simulink model "CM010A_GmT1xxMcuCfg"  (R2013b)
settings: Solver=FixedStepDiscrete  SolverMode=SingleTasking  StartTime=0.0  StopTime=0.05  RelTol=1e-3
undefined symbols (not defined in the file): BATTVLTGSCAGFAC_ULS_F32, BATTVLTGSWD1SCAGFAC_ULS_F32, BATTVLTGSWD2SCAGFAC_ULS_F32, sigbuilder_block
libraries: CM010A_GmT1xxMcuCfg_ModelLibrary x68, simulink x31
(part 2 of 3)

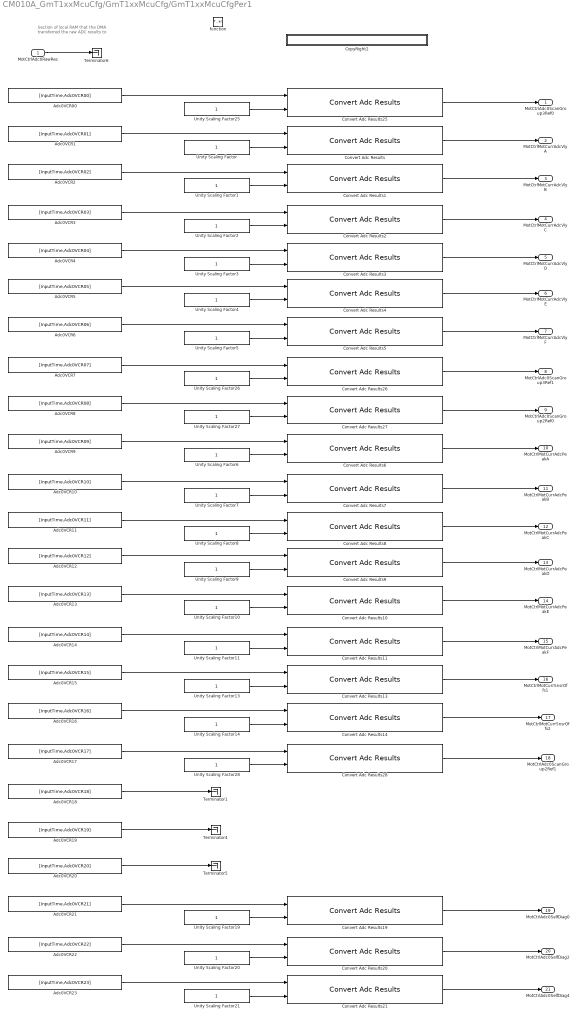
== system CM010A_GmT1xxMcuCfg/GmT1xxMcuCfg/GmT1xxMcuCfgPer1 ==
  note: Section of local RAM that the
      | DMA transferred the raw
      | ADC results to
  MotCtrlAdc0RawRes : Inport
  function : TriggerPort  TriggerType=function-call
  Adc0VCR00 : FromWorkspace  RequirementInfo={'linktype_rmi_doors' '000089ae (/ESG Group/FDD Module Requirements/ES FDDs/ES-50A DigMSB Allegro A1331)' '#ES50A_543' 'true' '3.3.2.2.0-1 The DigMSB Allegro 1331 Function shall indicate the integrity' '' } %GIDa_3972507b_7f96_4457_a8c5_9a064fa93529  VariableName=[InputTime,Adc0VCR00]  Interpolate=off  OutputAfterFinalValue=Holding final value
  Adc0VCR1 : FromWorkspace  RequirementInfo={'linktype_rmi_doors' '000089ae (/ESG Group/FDD Module Requirements/ES FDDs/ES-50A DigMSB Allegro A1331)' '#ES50A_543' 'true' '3.3.2.2.0-1 The DigMSB Allegro 1331 Function shall indicate the integrity' '' } %GIDa_8df7c0a1_9c18_4830_b8c1_52194c851c06  VariableName=[InputTime,Adc0VCR01]  Interpolate=off  OutputAfterFinalValue=Holding final value
  Adc0VCR10 : FromWorkspace  RequirementInfo={'linktype_rmi_doors' '000089ae (/ESG Group/FDD Module Requirements/ES FDDs/ES-50A DigMSB Allegro A1331)' '#ES50A_543' 'true' '3.3.2.2.0-1 The DigMSB Allegro 1331 Function shall indicate the integrity' '' } %GIDa_ced24115_ee0e_48d7_a1c5_ed88c1ec89e4  VariableName=[InputTime,Adc0VCR10]  Interpolate=off  OutputAfterFinalValue=Holding final value
  Adc0VCR11 : FromWorkspace  RequirementInfo={'linktype_rmi_doors' '000089ae (/ESG Group/FDD Module Requirements/ES FDDs/ES-50A DigMSB Allegro A1331)' '#ES50A_543' 'true' '3.3.2.2.0-1 The DigMSB Allegro 1331 Function shall indicate the integrity' '' } %GIDa_db2b065f_31fb_41aa_814a_e5cf8b57cff8  VariableName=[InputTime,Adc0VCR11]  Interpolate=off  OutputAfterFinalValue=Holding final value
  Adc0VCR12 : FromWorkspace  RequirementInfo={'linktype_rmi_doors' '000089ae (/ESG Group/FDD Module Requirements/ES FDDs/ES-50A DigMSB Allegro A1331)' '#ES50A_543' 'true' '3.3.2.2.0-1 The DigMSB Allegro 1331 Function shall indicate the integrity' '' } %GIDa_d2596e36_6e68_4a9e_ad4d_131e4edbf304  VariableName=[InputTime,Adc0VCR12]  Interpolate=off  OutputAfterFinalValue=Holding final value
  Adc0VCR13 : FromWorkspace  RequirementInfo={'linktype_rmi_doors' '000089ae (/ESG Group/FDD Module Requirements/ES FDDs/ES-50A DigMSB Allegro A1331)' '#ES50A_543' 'true' '3.3.2.2.0-1 The DigMSB Allegro 1331 Function shall indicate the integrity' '' } %GIDa_588422b8_9a00_4d95_845d_3e9dda5825e6  VariableName=[InputTime,Adc0VCR13]  Interpolate=off  OutputAfterFinalValue=Holding final value
  Adc0VCR14 : FromWorkspace  RequirementInfo={'linktype_rmi_doors' '000089ae (/ESG Group/FDD Module Requirements/ES FDDs/ES-50A DigMSB Allegro A1331)' '#ES50A_543' 'true' '3.3.2.2.0-1 The DigMSB Allegro 1331 Function shall indicate the integrity' '' } %GIDa_7f782811_0c4f_4bde_8d07_b52392360608  VariableName=[InputTime,Adc0VCR14]  Interpolate=off  OutputAfterFinalValue=Holding final value
  Adc0VCR15 : FromWorkspace  RequirementInfo={'linktype_rmi_doors' '000089ae (/ESG Group/FDD Module Requirements/ES FDDs/ES-50A DigMSB Allegro A1331)' '#ES50A_543' 'true' '3.3.2.2.0-1 The DigMSB Allegro 1331 Function shall indicate the integrity' '' } %GIDa_e774656f_bc2d_46bf_a587_e8a39f34598c  VariableName=[InputTime,Adc0VCR15]  Interpolate=off  OutputAfterFinalValue=Holding final value
  Adc0VCR16 : FromWorkspace  RequirementInfo={'linktype_rmi_doors' '000089ae (/ESG Group/FDD Module Requirements/ES FDDs/ES-50A DigMSB Allegro A1331)' '#ES50A_543' 'true' '3.3.2.2.0-1 The DigMSB Allegro 1331 Function shall indicate the integrity' '' } %GIDa_f44d6d24_48ad_4518_886b_ff8438f6312a  VariableName=[InputTime,Adc0VCR16]  Interpolate=off  OutputAfterFinalValue=Holding final value
  Adc0VCR17 : FromWorkspace  RequirementInfo={'linktype_rmi_doors' '000089ae (/ESG Group/FDD Module Requirements/ES FDDs/ES-50A DigMSB Allegro A1331)' '#ES50A_543' 'true' '3.3.2.2.0-1 The DigMSB Allegro 1331 Function shall indicate the integrity' '' } %GIDa_4675bda8_e067_4190_b347_8310ec6ff6c1  VariableName=[InputTime,Adc0VCR17]  Interpolate=off  OutputAfterFinalValue=Holding final value
  Adc0VCR18 : FromWorkspace  RequirementInfo={'linktype_rmi_doors' '000089ae (/ESG Group/FDD Module Requirements/ES FDDs/ES-50A DigMSB Allegro A1331)' '#ES50A_543' 'true' '3.3.2.2.0-1 The DigMSB Allegro 1331 Function shall indicate the integrity' '' } %GIDa_5aa89b95_9bd8_4248_9c0f_b5e881e1f776  VariableName=[InputTime,Adc0VCR18]  Interpolate=off  OutputAfterFinalValue=Holding final value
  Adc0VCR19 : FromWorkspace  RequirementInfo={'linktype_rmi_doors' '000089ae (/ESG Group/FDD Module Requirements/ES FDDs/ES-50A DigMSB Allegro A1331)' '#ES50A_543' 'true' '3.3.2.2.0-1 The DigMSB Allegro 1331 Function shall indicate the integrity' '' } %GIDa_d11aca7d_abc9_46a3_9261_b33926c9d20c  VariableName=[InputTime,Adc0VCR19]  Interpolate=off  OutputAfterFinalValue=Holding final value
  Adc0VCR2 : FromWorkspace  RequirementInfo={'linktype_rmi_doors' '000089ae (/ESG Group/FDD Module Requirements/ES FDDs/ES-50A DigMSB Allegro A1331)' '#ES50A_543' 'true' '3.3.2.2.0-1 The DigMSB Allegro 1331 Function shall indicate the integrity' '' } %GIDa_f6b758eb_17b3_4646_850a_50046f5107be  VariableName=[InputTime,Adc0VCR02]  Interpolate=off  OutputAfterFinalValue=Holding final value
  Adc0VCR20 : FromWorkspace  RequirementInfo={'linktype_rmi_doors' '000089ae (/ESG Group/FDD Module Requirements/ES FDDs/ES-50A DigMSB Allegro A1331)' '#ES50A_543' 'true' '3.3.2.2.0-1 The DigMSB Allegro 1331 Function shall indicate the integrity' '' } %GIDa_43dd3eb4_cf09_4920_adef_b45211e1cdfd  VariableName=[InputTime,Adc0VCR20]  Interpolate=off  OutputAfterFinalValue=Holding final value
  Adc0VCR21 : FromWorkspace  RequirementInfo={'linktype_rmi_doors' '000089ae (/ESG Group/FDD Module Requirements/ES FDDs/ES-50A DigMSB Allegro A1331)' '#ES50A_543' 'true' '3.3.2.2.0-1 The DigMSB Allegro 1331 Function shall indicate the integrity' '' } %GIDa_6a9825af_16e5_42b4_afa2_2084b93d0a1b  VariableName=[InputTime,Adc0VCR21]  Interpolate=off  OutputAfterFinalValue=Holding final value
  Adc0VCR22 : FromWorkspace  RequirementInfo={'linktype_rmi_doors' '000089ae (/ESG Group/FDD Module Requirements/ES FDDs/ES-50A DigMSB Allegro A1331)' '#ES50A_543' 'true' '3.3.2.2.0-1 The DigMSB Allegro 1331 Function shall indicate the integrity' '' } %GIDa_29a8826e_1cf3_4183_be72_0450154b9da2  VariableName=[InputTime,Adc0VCR22]  Interpolate=off  OutputAfterFinalValue=Holding final value
  Adc0VCR23 : FromWorkspace  RequirementInfo={'linktype_rmi_doors' '000089ae (/ESG Group/FDD Module Requirements/ES FDDs/ES-50A DigMSB Allegro A1331)' '#ES50A_543' 'true' '3.3.2.2.0-1 The DigMSB Allegro 1331 Function shall indicate the integrity' '' } %GIDa_8d461b89_add0_42d0_84ba_8109d18c3aa6  VariableName=[InputTime,Adc0VCR23]  Interpolate=off  OutputAfterFinalValue=Holding final value
  Adc0VCR3 : FromWorkspace  RequirementInfo={'linktype_rmi_doors' '000089ae (/ESG Group/FDD Module Requirements/ES FDDs/ES-50A DigMSB Allegro A1331)' '#ES50A_543' 'true' '3.3.2.2.0-1 The DigMSB Allegro 1331 Function shall indicate the integrity' '' } %GIDa_7f5e4bfd_0dc0_4fd2_91a2_992d3fd35db3  VariableName=[InputTime,Adc0VCR03]  Interpolate=off  OutputAfterFinalValue=Holding final value
  Adc0VCR4 : FromWorkspace  RequirementInfo={'linktype_rmi_doors' '000089ae (/ESG Group/FDD Module Requirements/ES FDDs/ES-50A DigMSB Allegro A1331)' '#ES50A_543' 'true' '3.3.2.2.0-1 The DigMSB Allegro 1331 Function shall indicate the integrity' '' } %GIDa_65871648_6683_4b6d_aff0_bffed2640892  VariableName=[InputTime,Adc0VCR04]  Interpolate=off  OutputAfterFinalValue=Holding final value
  Adc0VCR5 : FromWorkspace  RequirementInfo={'linktype_rmi_doors' '000089ae (/ESG Group/FDD Module Requirements/ES FDDs/ES-50A DigMSB Allegro A1331)' '#ES50A_543' 'true' '3.3.2.2.0-1 The DigMSB Allegro 1331 Function shall indicate the integrity' '' } %GIDa_516afef0_9b4d_432f_89dd_5f746eb09d49  VariableName=[InputTime,Adc0VCR05]  Interpolate=off  OutputAfterFinalValue=Holding final value
  Adc0VCR6 : FromWorkspace  RequirementInfo={'linktype_rmi_doors' '000089ae (/ESG Group/FDD Module Requirements/ES FDDs/ES-50A DigMSB Allegro A1331)' '#ES50A_543' 'true' '3.3.2.2.0-1 The DigMSB Allegro 1331 Function shall indicate the integrity' '' } %GIDa_384fee31_75ed_46f0_a695_7bc76fa48fd4  VariableName=[InputTime,Adc0VCR06]  Interpolate=off  OutputAfterFinalValue=Holding final value
  Adc0VCR7 : FromWorkspace  RequirementInfo={'linktype_rmi_doors' '000089ae (/ESG Group/FDD Module Requirements/ES FDDs/ES-50A DigMSB Allegro A1331)' '#ES50A_543' 'true' '3.3.2.2.0-1 The DigMSB Allegro 1331 Function shall indicate the integrity' '' } %GIDa_8c377a38_d7bd_42ca_a29f_4b53229cfff5  VariableName=[InputTime,Adc0VCR07]  Interpolate=off  OutputAfterFinalValue=Holding final value
  Adc0VCR8 : FromWorkspace  RequirementInfo={'linktype_rmi_doors' '000089ae (/ESG Group/FDD Module Requirements/ES FDDs/ES-50A DigMSB Allegro A1331)' '#ES50A_543' 'true' '3.3.2.2.0-1 The DigMSB Allegro 1331 Function shall indicate the integrity' '' } %GIDa_dae074de_385b_4abf_a24d_4693de33c827  VariableName=[InputTime,Adc0VCR08]  Interpolate=off  OutputAfterFinalValue=Holding final value
  Adc0VCR9 : FromWorkspace  RequirementInfo={'linktype_rmi_doors' '000089ae (/ESG Group/FDD Module Requirements/ES FDDs/ES-50A DigMSB Allegro A1331)' '#ES50A_543' 'true' '3.3.2.2.0-1 The DigMSB Allegro 1331 Function shall indicate the integrity' '' } %GIDa_c1adce1a_ec60_4755_95aa_f8dbf63dfb59  VariableName=[InputTime,Adc0VCR09]  Interpolate=off  OutputAfterFinalValue=Holding final value
  Convert Adc Results{,1..11,13..14,19..21,25..28} (21 alike) : CM010A_GmT1xxMcuCfg_ModelLibrary/Convert Adc Results
  CopyRight2 : Subsystem  Description=|  mask(Copyright Information){none=on}
      | Copyright info block.                                               
      |                                                                     
      | Place copyright information at the top of every subsystem in design.
      mask prompts: none "No parameters"
      mask help: Place copyright information at the top of every subsystem in design.
      mask Display:
      | NxtrConf = 'Nexteer Confidential';
      | 
      | sys = bdroot; %handle for the current model ("system")
      | first = get_param(sys,'Created');
      | first = first(end-3:end);  %year is last four digits
      | 
      | last = get_param(sys,'LastModifiedDate');
      | if isempty(last)
      |     last = datestr(now,'yyyy');
      | else
      |     last = last(end-3:end);
      | end
      | 
      | if strcmp(first,last)
      |     fprintf('%s -- Copyright %s Nexteer',NxtrConf,first)
      | else
      |     fprintf('%s -- %s%s- %s Nexteer',NxtrConf,char(169),first,last)
      | end
  Terminator{1,4..6} (4 alike) : Terminator
  Unity Scaling Factor{,1..11,13..14,19..21,25..28} (21 alike) : Constant  OutDataTypeStr=single
  MotCtrlAdc0ScanGroup3Ref0 : Outport
  MotCtrlMotCurrAdcVlyA : Outport  Port=2
  MotCtrlMotCurrAdcVlyB : Outport  Port=3
  MotCtrlMotCurrAdcVlyC : Outport  Port=4
  MotCtrlMotCurrAdcVlyD : Outport  Port=5
  MotCtrlMotCurrAdcVlyE : Outport  Port=6
  MotCtrlMotCurrAdcVlyF : Outport  Port=7
  MotCtrlAdc0ScanGroup3Ref1 : Outport  Port=8
  MotCtrlAdc0ScanGroup2Ref0 : Outport  Port=9
  MotCtrlMotCurrAdcPeakA : Outport  Port=10
  MotCtrlMotCurrAdcPeakB : Outport  Port=11
  MotCtrlMotCurrAdcPeakC : Outport  Port=12
  MotCtrlMotCurrAdcPeakD : Outport  Port=13
  MotCtrlMotCurrAdcPeakE : Outport  Port=14
  MotCtrlMotCurrAdcPeakF : Outport  Port=15
  MotCtrlMotCurrSnsrOffs1 : Outport  Port=16
  MotCtrlMotCurrSnsrOffs2 : Outport  Port=17
  MotCtrlAdc0ScanGroup2Ref1 : Outport  Port=18
  MotCtrlAdc0SelfDiag0 : Outport  Port=19
  MotCtrlAdc0SelfDiag2 : Outport  Port=20
  MotCtrlAdc0SelfDiag4 : Outport  Port=21
  wires:
  Unity Scaling Factor/1 -> Convert Adc Results/2
  Unity Scaling Factor1/1 -> Convert Adc Results1/2
  Unity Scaling Factor2/1 -> Convert Adc Results2/2
  Unity Scaling Factor3/1 -> Convert Adc Results3/2
  Unity Scaling Factor4/1 -> Convert Adc Results4/2
  Unity Scaling Factor5/1 -> Convert Adc Results5/2
  Unity Scaling Factor6/1 -> Convert Adc Results6/2
  Unity Scaling Factor7/1 -> Convert Adc Results7/2
  Unity Scaling Factor8/1 -> Convert Adc Results8/2
  Unity Scaling Factor9/1 -> Convert Adc Results9/2
  Unity Scaling Factor10/1 -> Convert Adc Results10/2
  Unity Scaling Factor11/1 -> Convert Adc Results11/2
  Unity Scaling Factor13/1 -> Convert Adc Results13/2
  Unity Scaling Factor14/1 -> Convert Adc Results14/2
  Adc0VCR21/1 -> Convert Adc Results19/1
  Unity Scaling Factor19/1 -> Convert Adc Results19/2
  Adc0VCR22/1 -> Convert Adc Results20/1
  Unity Scaling Factor20/1 -> Convert Adc Results20/2
  Adc0VCR23/1 -> Convert Adc Results21/1
  Unity Scaling Factor21/1 -> Convert Adc Results21/2
  Convert Adc Results2/1 -> MotCtrlMotCurrAdcVlyC/1
  Convert Adc Results3/1 -> MotCtrlMotCurrAdcVlyD/1
  Convert Adc Results4/1 -> MotCtrlMotCurrAdcVlyE/1
  Convert Adc Results5/1 -> MotCtrlMotCurrAdcVlyF/1
  Convert Adc Results6/1 -> MotCtrlMotCurrAdcPeakA/1
  Convert Adc Results7/1 -> MotCtrlMotCurrAdcPeakB/1
  Convert Adc Results8/1 -> MotCtrlMotCurrAdcPeakC/1
  Convert Adc Results9/1 -> MotCtrlMotCurrAdcPeakD/1
  Convert Adc Results10/1 -> MotCtrlMotCurrAdcPeakE/1
  Convert Adc Results11/1 -> MotCtrlMotCurrAdcPeakF/1
  Convert Adc Results13/1 -> MotCtrlMotCurrSnsrOffs1/1
  Convert Adc Results14/1 -> MotCtrlMotCurrSnsrOffs2/1
  Convert Adc Results19/1 -> MotCtrlAdc0SelfDiag0/1
  Convert Adc Results20/1 -> MotCtrlAdc0SelfDiag2/1
  Convert Adc Results21/1 -> MotCtrlAdc0SelfDiag4/1
  Adc0VCR20/1 -> Terminator5/1
  Adc0VCR19/1 -> Terminator4/1
  MotCtrlAdc0RawRes/1 -> Terminator6/1
  Unity Scaling Factor25/1 -> Convert Adc Results25/2
  Convert Adc Results25/1 -> MotCtrlAdc0ScanGroup3Ref0/1
  Unity Scaling Factor26/1 -> Convert Adc Results26/2
  Convert Adc Results26/1 -> MotCtrlAdc0ScanGroup3Ref1/1
  Unity Scaling Factor27/1 -> Convert Adc Results27/2
  Convert Adc Results27/1 -> MotCtrlAdc0ScanGroup2Ref0/1
  Unity Scaling Factor28/1 -> Convert Adc Results28/2
  Convert Adc Results28/1 -> MotCtrlAdc0ScanGroup2Ref1/1
  Adc0VCR1/1 -> Convert Adc Results/1
  Adc0VCR7/1 -> Convert Adc Results26/1
  Adc0VCR8/1 -> Convert Adc Results27/1
  Adc0VCR00/1 -> Convert Adc Results25/1
  Convert Adc Results1/1 -> MotCtrlMotCurrAdcVlyB/1
  Convert Adc Results/1 -> MotCtrlMotCurrAdcVlyA/1
  Adc0VCR14/1 -> Convert Adc Results11/1
  Adc0VCR13/1 -> Convert Adc Results10/1
  Adc0VCR12/1 -> Convert Adc Results9/1
  Adc0VCR11/1 -> Convert Adc Results8/1
  Adc0VCR10/1 -> Convert Adc Results7/1
  Adc0VCR9/1 -> Convert Adc Results6/1
  Adc0VCR6/1 -> Convert Adc Results5/1
  Adc0VCR5/1 -> Convert Adc Results4/1
  Adc0VCR4/1 -> Convert Adc Results3/1
  Adc0VCR3/1 -> Convert Adc Results2/1
  Adc0VCR2/1 -> Convert Adc Results1/1
  Adc0VCR15/1 -> Convert Adc Results13/1
  Adc0VCR16/1 -> Convert Adc Results14/1
  Adc0VCR17/1 -> Convert Adc Results28/1
  Adc0VCR18/1 -> Terminator1/1

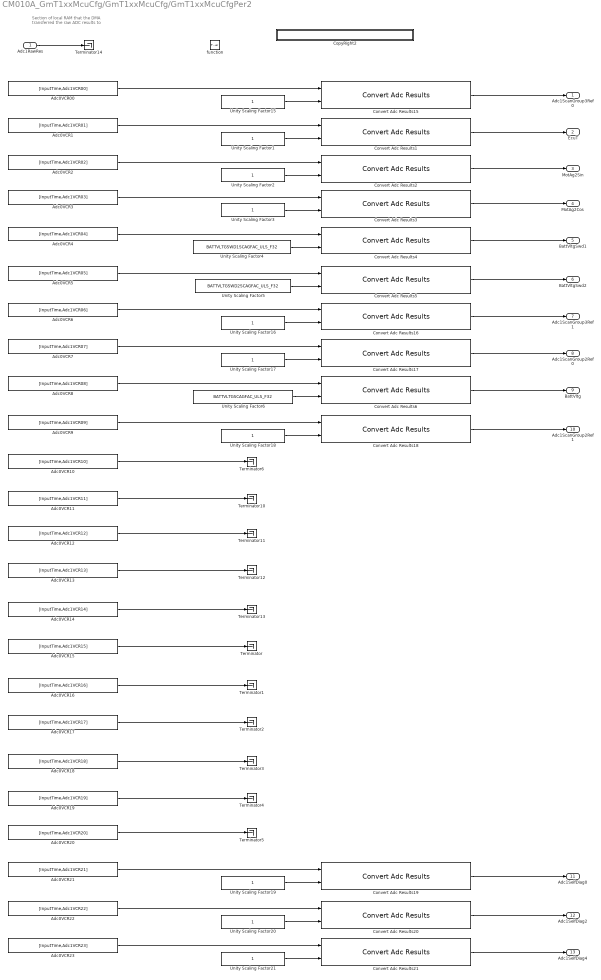
== system CM010A_GmT1xxMcuCfg/GmT1xxMcuCfg/GmT1xxMcuCfgPer2 ==
  note: Section of local RAM that the
      | DMA transferred the raw
      | ADC results to
  Adc1RawRes : Inport
  function : TriggerPort  TriggerType=function-call
  Adc0VCR00 : FromWorkspace  RequirementInfo={'linktype_rmi_doors' '000089ae (/ESG Group/FDD Module Requirements/ES FDDs/ES-50A DigMSB Allegro A1331)' '#ES50A_543' 'true' '3.3.2.2.0-1 The DigMSB Allegro 1331 Function shall indicate the integrity' '' } %GIDa_56da86a8_cfa1_4b5f_b5e2_87394d82ad94  VariableName=[InputTime,Adc1VCR00]  Interpolate=off  OutputAfterFinalValue=Holding final value
  Adc0VCR1 : FromWorkspace  RequirementInfo={'linktype_rmi_doors' '000089ae (/ESG Group/FDD Module Requirements/ES FDDs/ES-50A DigMSB Allegro A1331)' '#ES50A_543' 'true' '3.3.2.2.0-1 The DigMSB Allegro 1331 Function shall indicate the integrity' '' } %GIDa_45c25bac_2c08_4aa3_a2d9_7c2ba87e4875  VariableName=[InputTime,Adc1VCR01]  Interpolate=off  OutputAfterFinalValue=Holding final value
  Adc0VCR10 : FromWorkspace  RequirementInfo={'linktype_rmi_doors' '000089ae (/ESG Group/FDD Module Requirements/ES FDDs/ES-50A DigMSB Allegro A1331)' '#ES50A_543' 'true' '3.3.2.2.0-1 The DigMSB Allegro 1331 Function shall indicate the integrity' '' } %GIDa_a6c55da2_28d1_43ef_b684_2673549cd623  VariableName=[InputTime,Adc1VCR10]  Interpolate=off  OutputAfterFinalValue=Holding final value
  Adc0VCR11 : FromWorkspace  RequirementInfo={'linktype_rmi_doors' '000089ae (/ESG Group/FDD Module Requirements/ES FDDs/ES-50A DigMSB Allegro A1331)' '#ES50A_543' 'true' '3.3.2.2.0-1 The DigMSB Allegro 1331 Function shall indicate the integrity' '' } %GIDa_c0e95f11_1daa_41de_b911_2a845480a7e4  VariableName=[InputTime,Adc1VCR11]  Interpolate=off  OutputAfterFinalValue=Holding final value
  Adc0VCR12 : FromWorkspace  RequirementInfo={'linktype_rmi_doors' '000089ae (/ESG Group/FDD Module Requirements/ES FDDs/ES-50A DigMSB Allegro A1331)' '#ES50A_543' 'true' '3.3.2.2.0-1 The DigMSB Allegro 1331 Function shall indicate the integrity' '' } %GIDa_5159a0ec_9e6f_46a5_bdcf_4d54449781c2  VariableName=[InputTime,Adc1VCR12]  Interpolate=off  OutputAfterFinalValue=Holding final value
  Adc0VCR13 : FromWorkspace  RequirementInfo={'linktype_rmi_doors' '000089ae (/ESG Group/FDD Module Requirements/ES FDDs/ES-50A DigMSB Allegro A1331)' '#ES50A_543' 'true' '3.3.2.2.0-1 The DigMSB Allegro 1331 Function shall indicate the integrity' '' } %GIDa_15b636da_7e99_43f2_bc55_3ecf242a137a  VariableName=[InputTime,Adc1VCR13]  Interpolate=off  OutputAfterFinalValue=Holding final value
  Adc0VCR14 : FromWorkspace  RequirementInfo={'linktype_rmi_doors' '000089ae (/ESG Group/FDD Module Requirements/ES FDDs/ES-50A DigMSB Allegro A1331)' '#ES50A_543' 'true' '3.3.2.2.0-1 The DigMSB Allegro 1331 Function shall indicate the integrity' '' } %GIDa_41e44980_6a48_4f6f_ab09_f9a0a5ff76cb  VariableName=[InputTime,Adc1VCR14]  Interpolate=off  OutputAfterFinalValue=Holding final value
  Adc0VCR15 : FromWorkspace  RequirementInfo={'linktype_rmi_doors' '000089ae (/ESG Group/FDD Module Requirements/ES FDDs/ES-50A DigMSB Allegro A1331)' '#ES50A_543' 'true' '3.3.2.2.0-1 The DigMSB Allegro 1331 Function shall indicate the integrity' '' } %GIDa_6a220150_fa15_47f5_b5f0_ba4b8132f148  VariableName=[InputTime,Adc1VCR15]  Interpolate=off  OutputAfterFinalValue=Holding final value
  Adc0VCR16 : FromWorkspace  RequirementInfo={'linktype_rmi_doors' '000089ae (/ESG Group/FDD Module Requirements/ES FDDs/ES-50A DigMSB Allegro A1331)' '#ES50A_543' 'true' '3.3.2.2.0-1 The DigMSB Allegro 1331 Function shall indicate the integrity' '' } %GIDa_e9f8c7af_0d13_4e13_b004_7a3aca79a10c  VariableName=[InputTime,Adc1VCR16]  Interpolate=off  OutputAfterFinalValue=Holding final value
  Adc0VCR17 : FromWorkspace  RequirementInfo={'linktype_rmi_doors' '000089ae (/ESG Group/FDD Module Requirements/ES FDDs/ES-50A DigMSB Allegro A1331)' '#ES50A_543' 'true' '3.3.2.2.0-1 The DigMSB Allegro 1331 Function shall indicate the integrity' '' } %GIDa_da51fb6d_e8c6_4c04_896b_631b85f822ab  VariableName=[InputTime,Adc1VCR17]  Interpolate=off  OutputAfterFinalValue=Holding final value
  Adc0VCR18 : FromWorkspace  RequirementInfo={'linktype_rmi_doors' '000089ae (/ESG Group/FDD Module Requirements/ES FDDs/ES-50A DigMSB Allegro A1331)' '#ES50A_543' 'true' '3.3.2.2.0-1 The DigMSB Allegro 1331 Function shall indicate the integrity' '' } %GIDa_eec1ee63_0ee0_4a98_a9ce_383d28f4f160  VariableName=[InputTime,Adc1VCR18]  Interpolate=off  OutputAfterFinalValue=Holding final value
  Adc0VCR19 : FromWorkspace  RequirementInfo={'linktype_rmi_doors' '000089ae (/ESG Group/FDD Module Requirements/ES FDDs/ES-50A DigMSB Allegro A1331)' '#ES50A_543' 'true' '3.3.2.2.0-1 The DigMSB Allegro 1331 Function shall indicate the integrity' '' } %GIDa_4061305a_2b96_47f1_9f04_00a22d375f8e  VariableName=[InputTime,Adc1VCR19]  Interpolate=off  OutputAfterFinalValue=Holding final value
  Adc0VCR2 : FromWorkspace  RequirementInfo={'linktype_rmi_doors' '000089ae (/ESG Group/FDD Module Requirements/ES FDDs/ES-50A DigMSB Allegro A1331)' '#ES50A_543' 'true' '3.3.2.2.0-1 The DigMSB Allegro 1331 Function shall indicate the integrity' '' } %GIDa_86007c37_1225_4ae0_8eed_a0b71d9b6c1c  VariableName=[InputTime,Adc1VCR02]  Interpolate=off  OutputAfterFinalValue=Holding final value
  Adc0VCR20 : FromWorkspace  RequirementInfo={'linktype_rmi_doors' '000089ae (/ESG Group/FDD Module Requirements/ES FDDs/ES-50A DigMSB Allegro A1331)' '#ES50A_543' 'true' '3.3.2.2.0-1 The DigMSB Allegro 1331 Function shall indicate the integrity' '' } %GIDa_330842db_6118_4db4_a002_0c8a20c8d852  VariableName=[InputTime,Adc1VCR20]  Interpolate=off  OutputAfterFinalValue=Holding final value
  Adc0VCR21 : FromWorkspace  RequirementInfo={'linktype_rmi_doors' '000089ae (/ESG Group/FDD Module Requirements/ES FDDs/ES-50A DigMSB Allegro A1331)' '#ES50A_543' 'true' '3.3.2.2.0-1 The DigMSB Allegro 1331 Function shall indicate the integrity' '' } %GIDa_3f089c77_bb2e_43f1_a982_c2c6f5ee80ef  VariableName=[InputTime,Adc1VCR21]  Interpolate=off  OutputAfterFinalValue=Holding final value
  Adc0VCR22 : FromWorkspace  RequirementInfo={'linktype_rmi_doors' '000089ae (/ESG Group/FDD Module Requirements/ES FDDs/ES-50A DigMSB Allegro A1331)' '#ES50A_543' 'true' '3.3.2.2.0-1 The DigMSB Allegro 1331 Function shall indicate the integrity' '' } %GIDa_74202af4_fd64_46fc_877a_7595b0e6817b  VariableName=[InputTime,Adc1VCR22]  Interpolate=off  OutputAfterFinalValue=Holding final value
  Adc0VCR23 : FromWorkspace  RequirementInfo={'linktype_rmi_doors' '000089ae (/ESG Group/FDD Module Requirements/ES FDDs/ES-50A DigMSB Allegro A1331)' '#ES50A_543' 'true' '3.3.2.2.0-1 The DigMSB Allegro 1331 Function shall indicate the integrity' '' } %GIDa_c2dd4636_4e0c_4eab_b443_996957062fe5  VariableName=[InputTime,Adc1VCR23]  Interpolate=off  OutputAfterFinalValue=Holding final value
  Adc0VCR3 : FromWorkspace  RequirementInfo={'linktype_rmi_doors' '000089ae (/ESG Group/FDD Module Requirements/ES FDDs/ES-50A DigMSB Allegro A1331)' '#ES50A_543' 'true' '3.3.2.2.0-1 The DigMSB Allegro 1331 Function shall indicate the integrity' '' } %GIDa_936b2d12_7e67_4fae_b361_731c2ff5f612  VariableName=[InputTime,Adc1VCR03]  Interpolate=off  OutputAfterFinalValue=Holding final value
  Adc0VCR4 : FromWorkspace  RequirementInfo={'linktype_rmi_doors' '000089ae (/ESG Group/FDD Module Requirements/ES FDDs/ES-50A DigMSB Allegro A1331)' '#ES50A_543' 'true' '3.3.2.2.0-1 The DigMSB Allegro 1331 Function shall indicate the integrity' '' } %GIDa_ce1e89a7_8a5e_4eb4_aa7b_0e1018bda303  VariableName=[InputTime,Adc1VCR04]  Interpolate=off  OutputAfterFinalValue=Holding final value
  Adc0VCR5 : FromWorkspace  RequirementInfo={'linktype_rmi_doors' '000089ae (/ESG Group/FDD Module Requirements/ES FDDs/ES-50A DigMSB Allegro A1331)' '#ES50A_543' 'true' '3.3.2.2.0-1 The DigMSB Allegro 1331 Function shall indicate the integrity' '' } %GIDa_de583444_1531_4319_8a34_b0fc27c5d24a  VariableName=[InputTime,Adc1VCR05]  Interpolate=off  OutputAfterFinalValue=Holding final value
  Adc0VCR6 : FromWorkspace  RequirementInfo={'linktype_rmi_doors' '000089ae (/ESG Group/FDD Module Requirements/ES FDDs/ES-50A DigMSB Allegro A1331)' '#ES50A_543' 'true' '3.3.2.2.0-1 The DigMSB Allegro 1331 Function shall indicate the integrity' '' } %GIDa_afd121dc_4485_4963_938c_5a108d83f017  VariableName=[InputTime,Adc1VCR06]  Interpolate=off  OutputAfterFinalValue=Holding final value
  Adc0VCR7 : FromWorkspace  RequirementInfo={'linktype_rmi_doors' '000089ae (/ESG Group/FDD Module Requirements/ES FDDs/ES-50A DigMSB Allegro A1331)' '#ES50A_543' 'true' '3.3.2.2.0-1 The DigMSB Allegro 1331 Function shall indicate the integrity' '' } %GIDa_9e7f179a_dc72_4f49_af61_04471e44937d  VariableName=[InputTime,Adc1VCR07]  Interpolate=off  OutputAfterFinalValue=Holding final value
  Adc0VCR8 : FromWorkspace  RequirementInfo={'linktype_rmi_doors' '000089ae (/ESG Group/FDD Module Requirements/ES FDDs/ES-50A DigMSB Allegro A1331)' '#ES50A_543' 'true' '3.3.2.2.0-1 The DigMSB Allegro 1331 Function shall indicate the integrity' '' } %GIDa_ef1ebe44_a6ab_4a0b_8802_ceced9e0f41d  VariableName=[InputTime,Adc1VCR08]  Interpolate=off  OutputAfterFinalValue=Holding final value
  Adc0VCR9 : FromWorkspace  RequirementInfo={'linktype_rmi_doors' '000089ae (/ESG Group/FDD Module Requirements/ES FDDs/ES-50A DigMSB Allegro A1331)' '#ES50A_543' 'true' '3.3.2.2.0-1 The DigMSB Allegro 1331 Function shall indicate the integrity' '' } %GIDa_1edf0447_598d_40e9_b4ea_decbaa9becbd  VariableName=[InputTime,Adc1VCR09]  Interpolate=off  OutputAfterFinalValue=Holding final value
  Convert Adc Results{1..6,15..21} (13 alike) : CM010A_GmT1xxMcuCfg_ModelLibrary/Convert Adc Results
  CopyRight2 : Subsystem  Description=|  mask(Copyright Information){none=on}
      | Copyright info block.                                               
      |                                                                     
      | Place copyright information at the top of every subsystem in design.
      mask prompts: none "No parameters"
      mask help: Place copyright information at the top of every subsystem in design.
      mask Display:
      | NxtrConf = 'Nexteer Confidential';
      | 
      | sys = bdroot; %handle for the current model ("system")
      | first = get_param(sys,'Created');
      | first = first(end-3:end);  %year is last four digits
      | 
      | last = get_param(sys,'LastModifiedDate');
      | if isempty(last)
      |     last = datestr(now,'yyyy');
      | else
      |     last = last(end-3:end);
      | end
      | 
      | if strcmp(first,last)
      |     fprintf('%s -- Copyright %s Nexteer',NxtrConf,first)
      | else
      |     fprintf('%s -- %s%s- %s Nexteer',NxtrConf,char(169),first,last)
      | end
  Terminator{,1..6,10..14} (12 alike) : Terminator
  Unity Scaling Factor{1..3,15..21} (10 alike) : Constant  OutDataTypeStr=single
  Unity Scaling Factor4 : Constant  Value=BATTVLTGSWD1SCAGFAC_ULS_F32  OutDataTypeStr=single
  Unity Scaling Factor5 : Constant  Value=BATTVLTGSWD2SCAGFAC_ULS_F32  OutDataTypeStr=single
  Unity Scaling Factor6 : Constant  Value=BATTVLTGSCAGFAC_ULS_F32  OutDataTypeStr=single
  Adc1ScanGroup3Ref0 : Outport
  EcuT : Outport  Port=2
  MotAg2Sin : Outport  Port=3
  MotAg2Cos : Outport  Port=4
  BattVltgSwd1 : Outport  Port=5
  BattVltgSwd2 : Outport  Port=6
  Adc1ScanGroup3Ref1 : Outport  Port=7
  Adc1ScanGroup2Ref0 : Outport  Port=8
  BattVltg : Outport  Port=9
  Adc1ScanGroup2Ref1 : Outport  Port=10
  Adc1SelfDiag0 : Outport  Port=11
  Adc1SelfDiag2 : Outport  Port=12
  Adc1SelfDiag4 : Outport  Port=13
  wires:
  Adc0VCR16/1 -> Terminator1/1
  Adc0VCR17/1 -> Terminator2/1
  Adc0VCR18/1 -> Terminator3/1
  Adc0VCR19/1 -> Terminator4/1
  Adc0VCR20/1 -> Terminator5/1
  Adc0VCR15/1 -> Terminator/1
  Convert Adc Results21/1 -> Adc1SelfDiag4/1
  Convert Adc Results20/1 -> Adc1SelfDiag2/1
  Convert Adc Results19/1 -> Adc1SelfDiag0/1
  Convert Adc Results6/1 -> BattVltg/1
  Convert Adc Results5/1 -> BattVltgSwd2/1
  Convert Adc Results4/1 -> BattVltgSwd1/1
  Convert Adc Results3/1 -> MotAg2Cos/1
  Convert Adc Results2/1 -> MotAg2Sin/1
  Convert Adc Results1/1 -> EcuT/1
  Unity Scaling Factor21/1 -> Convert Adc Results21/2
  Adc0VCR23/1 -> Convert Adc Results21/1
  Unity Scaling Factor20/1 -> Convert Adc Results20/2
  Adc0VCR22/1 -> Convert Adc Results20/1
  Unity Scaling Factor19/1 -> Convert Adc Results19/2
  Adc0VCR21/1 -> Convert Adc Results19/1
  Unity Scaling Factor6/1 -> Convert Adc Results6/2
  Unity Scaling Factor5/1 -> Convert Adc Results5/2
  Unity Scaling Factor4/1 -> Convert Adc Results4/2
  Unity Scaling Factor3/1 -> Convert Adc Results3/2
  Unity Scaling Factor2/1 -> Convert Adc Results2/2
  Unity Scaling Factor1/1 -> Convert Adc Results1/2
  Adc0VCR11/1 -> Terminator10/1
  Adc0VCR12/1 -> Terminator11/1
  Adc0VCR13/1 -> Terminator12/1
  Adc0VCR14/1 -> Terminator13/1
  Adc1RawRes/1 -> Terminator14/1
  Unity Scaling Factor15/1 -> Convert Adc Results15/2
  Convert Adc Results15/1 -> Adc1ScanGroup3Ref0/1
  Unity Scaling Factor16/1 -> Convert Adc Results16/2
  Convert Adc Results16/1 -> Adc1ScanGroup3Ref1/1
  Unity Scaling Factor17/1 -> Convert Adc Results17/2
  Convert Adc Results17/1 -> Adc1ScanGroup2Ref0/1
  Unity Scaling Factor18/1 -> Convert Adc Results18/2
  Convert Adc Results18/1 -> Adc1ScanGroup2Ref1/1
  Adc0VCR00/1 -> Convert Adc Results15/1
  Adc0VCR1/1 -> Convert Adc Results1/1
  Adc0VCR2/1 -> Convert Adc Results2/1
  Adc0VCR3/1 -> Convert Adc Results3/1
  Adc0VCR4/1 -> Convert Adc Results4/1
  Adc0VCR5/1 -> Convert Adc Results5/1
  Adc0VCR6/1 -> Convert Adc Results16/1
  Adc0VCR7/1 -> Convert Adc Results17/1
  Adc0VCR8/1 -> Convert Adc Results6/1
  Adc0VCR9/1 -> Convert Adc Results18/1
  Adc0VCR10/1 -> Terminator6/1

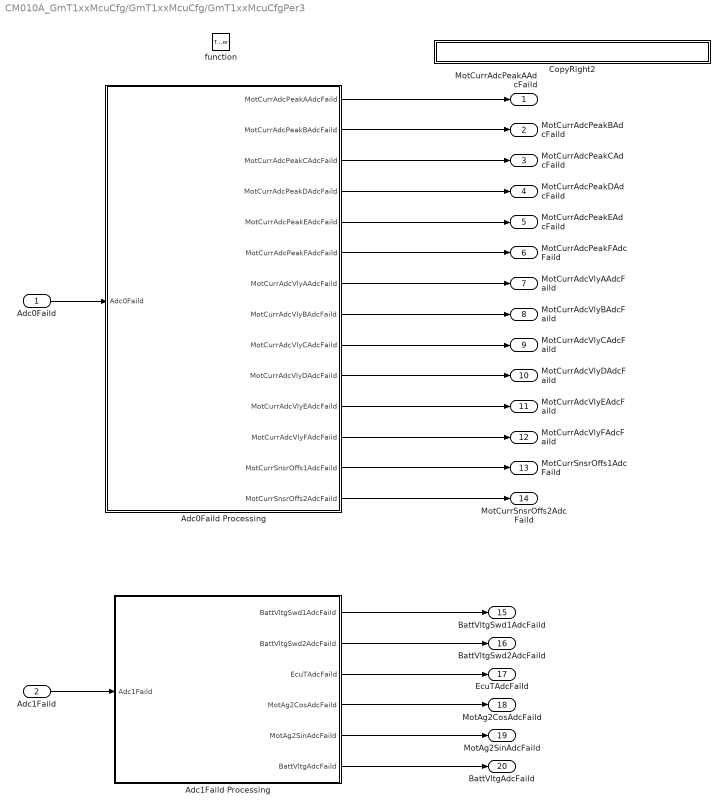
== system CM010A_GmT1xxMcuCfg/GmT1xxMcuCfg/GmT1xxMcuCfgPer3 ==
  Adc0Faild : Inport
  Adc1Faild : Inport  Port=2
  function : TriggerPort  TriggerType=function-call
  Adc0Faild Processing : Subsystem  TreatAsAtomicUnit=on
  Adc1Faild Processing : Subsystem  TreatAsAtomicUnit=on
  CopyRight2 : Subsystem  Description=|  mask(Copyright Information){none=on}
      | Copyright info block.                                               
      |                                                                     
      | Place copyright information at the top of every subsystem in design.
      mask prompts: none "No parameters"
      mask help: Place copyright information at the top of every subsystem in design.
      mask Display:
      | NxtrConf = 'Nexteer Confidential';
      | 
      | sys = bdroot; %handle for the current model ("system")
      | first = get_param(sys,'Created');
      | first = first(end-3:end);  %year is last four digits
      | 
      | last = get_param(sys,'LastModifiedDate');
      | if isempty(last)
      |     last = datestr(now,'yyyy');
      | else
      |     last = last(end-3:end);
      | end
      | 
      | if strcmp(first,last)
      |     fprintf('%s -- Copyright %s Nexteer',NxtrConf,first)
      | else
      |     fprintf('%s -- %s%s- %s Nexteer',NxtrConf,char(169),first,last)
      | end
  MotCurrAdcPeakAAdcFaild : Outport
  MotCurrAdcPeakBAdcFaild : Outport  Port=2
  MotCurrAdcPeakCAdcFaild : Outport  Port=3
  MotCurrAdcPeakDAdcFaild : Outport  Port=4
  MotCurrAdcPeakEAdcFaild : Outport  Port=5
  MotCurrAdcPeakFAdcFaild : Outport  Port=6
  MotCurrAdcVlyAAdcFaild : Outport  Port=7
  MotCurrAdcVlyBAdcFaild : Outport  Port=8
  MotCurrAdcVlyCAdcFaild : Outport  Port=9
  MotCurrAdcVlyDAdcFaild : Outport  Port=10
  MotCurrAdcVlyEAdcFaild : Outport  Port=11
  MotCurrAdcVlyFAdcFaild : Outport  Port=12
  MotCurrSnsrOffs1AdcFaild : Outport  Port=13
  MotCurrSnsrOffs2AdcFaild : Outport  Port=14
  BattVltgSwd1AdcFaild : Outport  Port=15
  BattVltgSwd2AdcFaild : Outport  Port=16
  EcuTAdcFaild : Outport  Port=17
  MotAg2CosAdcFaild : Outport  Port=18
  MotAg2SinAdcFaild : Outport  Port=19
  BattVltgAdcFaild : Outport  Port=20
  wires:
  Adc0Faild/1 -> Adc0Faild Processing/1(Adc0Faild)
  Adc0Faild Processing/1(MotCurrAdcPeakAAdcFaild) -> MotCurrAdcPeakAAdcFaild/1
  Adc0Faild Processing/2(MotCurrAdcPeakBAdcFaild) -> MotCurrAdcPeakBAdcFaild/1
  Adc0Faild Processing/3(MotCurrAdcPeakCAdcFaild) -> MotCurrAdcPeakCAdcFaild/1
  Adc0Faild Processing/4(MotCurrAdcPeakDAdcFaild) -> MotCurrAdcPeakDAdcFaild/1
  Adc0Faild Processing/5(MotCurrAdcPeakEAdcFaild) -> MotCurrAdcPeakEAdcFaild/1
  Adc0Faild Processing/6(MotCurrAdcPeakFAdcFaild) -> MotCurrAdcPeakFAdcFaild/1
  Adc0Faild Processing/7(MotCurrAdcVlyAAdcFaild) -> MotCurrAdcVlyAAdcFaild/1
  Adc0Faild Processing/8(MotCurrAdcVlyBAdcFaild) -> MotCurrAdcVlyBAdcFaild/1
  Adc0Faild Processing/9(MotCurrAdcVlyCAdcFaild) -> MotCurrAdcVlyCAdcFaild/1
  Adc0Faild Processing/10(MotCurrAdcVlyDAdcFaild) -> MotCurrAdcVlyDAdcFaild/1
  Adc0Faild Processing/11(MotCurrAdcVlyEAdcFaild) -> MotCurrAdcVlyEAdcFaild/1
  Adc0Faild Processing/12(MotCurrAdcVlyFAdcFaild) -> MotCurrAdcVlyFAdcFaild/1
  Adc0Faild Processing/13(MotCurrSnsrOffs1AdcFaild) -> MotCurrSnsrOffs1AdcFaild/1
  Adc0Faild Processing/14(MotCurrSnsrOffs2AdcFaild) -> MotCurrSnsrOffs2AdcFaild/1
  Adc1Faild/1 -> Adc1Faild Processing/1(Adc1Faild)
  Adc1Faild Processing/1(BattVltgSwd1AdcFaild) -> BattVltgSwd1AdcFaild/1
  Adc1Faild Processing/2(BattVltgSwd2AdcFaild) -> BattVltgSwd2AdcFaild/1
  Adc1Faild Processing/3(EcuTAdcFaild) -> EcuTAdcFaild/1
  Adc1Faild Processing/4(MotAg2CosAdcFaild) -> MotAg2CosAdcFaild/1
  Adc1Faild Processing/5(MotAg2SinAdcFaild) -> MotAg2SinAdcFaild/1
  Adc1Faild Processing/6(BattVltgAdcFaild) -> BattVltgAdcFaild/1

== system CM010A_GmT1xxMcuCfg/GmT1xxMcuCfg/GmT1xxMcuCfgInit1/CopyRight2 ==

== system CM010A_GmT1xxMcuCfg/GmT1xxMcuCfg/GmT1xxMcuCfgInit1/Register Initialization ==
  note: GmT1xxMcuCfg Configuration
      | Initialize the PIC2B registers from the following sources in the order listed:
      |
      |
      | 1. Run Adc0CfgAndUseInit1 - this means to run the AdcCfgInit function first before this init function, there is no client or server call
      | 2  Run Adc1CfgAndUseInit1 - this means to run the AdcCfgInit function first before this init function, there is no client or server call
      | 3. CM010A_GmT1xxMcuCfg_RegisterConfiguration.xlsm
      |     Order by row
  CopyRight2 : Subsystem  Description=|  mask(Copyright Information){none=on}
      | Copyright info block.                                               
      |                                                                     
      | Place copyright information at the top of every subsystem in design.
      mask prompts: none "No parameters"
      mask help: Place copyright information at the top of every subsystem in design.
      mask Display:
      | NxtrConf = 'Nexteer Confidential';
      | 
      | sys = bdroot; %handle for the current model ("system")
      | first = get_param(sys,'Created');
      | first = first(end-3:end);  %year is last four digits
      | 
      | last = get_param(sys,'LastModifiedDate');
      | if isempty(last)
      |     last = datestr(now,'yyyy');
      | else
      |     last = last(end-3:end);
      | end
      | 
      | if strcmp(first,last)
      |     fprintf('%s -- Copyright %s Nexteer',NxtrConf,first)
      | else
      |     fprintf('%s -- %s%s- %s Nexteer',NxtrConf,char(169),first,last)
      | end

== system CM010A_GmT1xxMcuCfg/GmT1xxMcuCfg/GmT1xxMcuCfgInit2/CopyRight2 ==

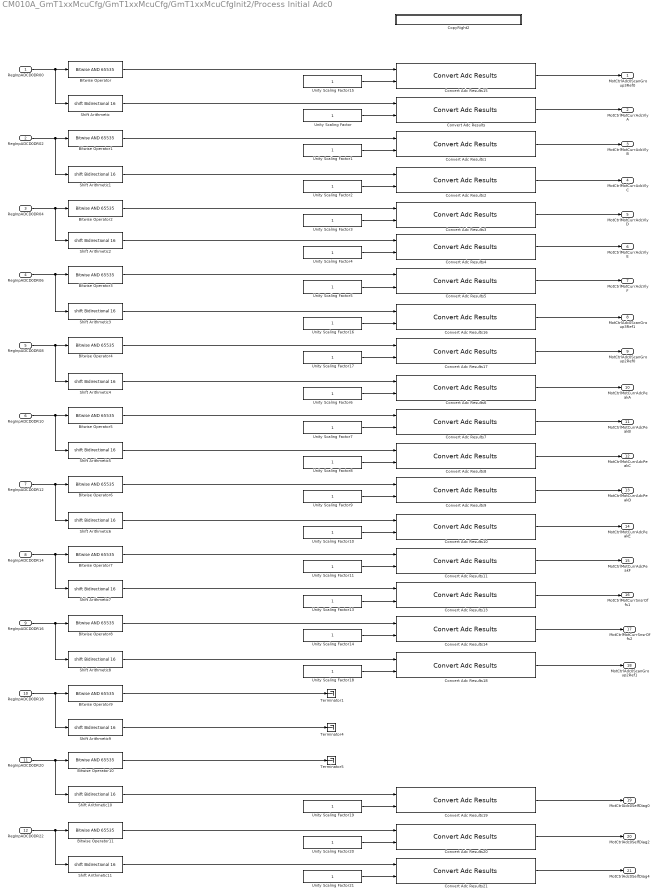
== system CM010A_GmT1xxMcuCfg/GmT1xxMcuCfg/GmT1xxMcuCfgInit2/Process Initial Adc0 ==
  RegInpADCD0DR00 : Inport  OutDataTypeStr=uint32
  RegInpADCD0DR02 : Inport  Port=2  OutDataTypeStr=uint32
  RegInpADCD0DR04 : Inport  Port=3  OutDataTypeStr=uint32
  RegInpADCD0DR06 : Inport  Port=4  OutDataTypeStr=uint32
  RegInpADCD0DR08 : Inport  Port=5  OutDataTypeStr=uint32
  RegInpADCD0DR10 : Inport  Port=6  OutDataTypeStr=uint32
  RegInpADCD0DR12 : Inport  Port=7  OutDataTypeStr=uint32
  RegInpADCD0DR14 : Inport  Port=8  OutDataTypeStr=uint32
  RegInpADCD0DR16 : Inport  Port=9  OutDataTypeStr=uint32
  RegInpADCD0DR18 : Inport  Port=10  OutDataTypeStr=uint32
  RegInpADCD0DR20 : Inport  Port=11  OutDataTypeStr=uint32
  RegInpADCD0DR22 : Inport  Port=12  OutDataTypeStr=uint32
  Bitwise Operator{,1..11} (12 alike) : simulink/Logic and Bit Operations/Bitwise Operator  logicop=AND  UseBitMask=on  BitMask=65535  BitMaskRealWorld=Stored Integer
  Convert Adc Results{,1..11,13..21} (21 alike) : CM010A_GmT1xxMcuCfg_ModelLibrary/Convert Adc Results
  CopyRight2 : Subsystem  Description=|  mask(Copyright Information){none=on}
      | Copyright info block.                                               
      |                                                                     
      | Place copyright information at the top of every subsystem in design.
      mask prompts: none "No parameters"
      mask help: Place copyright information at the top of every subsystem in design.
      mask Display:
      | NxtrConf = 'Nexteer Confidential';
      | 
      | sys = bdroot; %handle for the current model ("system")
      | first = get_param(sys,'Created');
      | first = first(end-3:end);  %year is last four digits
      | 
      | last = get_param(sys,'LastModifiedDate');
      | if isempty(last)
      |     last = datestr(now,'yyyy');
      | else
      |     last = last(end-3:end);
      | end
      | 
      | if strcmp(first,last)
      |     fprintf('%s -- Copyright %s Nexteer',NxtrConf,first)
      | else
      |     fprintf('%s -- %s%s- %s Nexteer',NxtrConf,char(169),first,last)
      | end
  Shift Arithmetic{,1..11} (12 alike) : ArithShift  BitShiftNumber=16
  Terminator1 : Terminator
  Terminator4 : Terminator
  Terminator5 : Terminator
  Unity Scaling Factor{,1..11,13..21} (21 alike) : Constant  OutDataTypeStr=single
  MotCtrlAdc0ScanGroup3Ref0 : Outport
  MotCtrlMotCurrAdcVlyA : Outport  Port=2
  MotCtrlMotCurrAdcVlyB : Outport  Port=3
  MotCtrlMotCurrAdcVlyC : Outport  Port=4
  MotCtrlMotCurrAdcVlyD : Outport  Port=5
  MotCtrlMotCurrAdcVlyE : Outport  Port=6
  MotCtrlMotCurrAdcVlyF : Outport  Port=7
  MotCtrlAdc0ScanGroup3Ref1 : Outport  Port=8
  MotCtrlAdc0ScanGroup2Ref0 : Outport  Port=9
  MotCtrlMotCurrAdcPeakA : Outport  Port=10
  MotCtrlMotCurrAdcPeakB : Outport  Port=11
  MotCtrlMotCurrAdcPeakC : Outport  Port=12
  MotCtrlMotCurrAdcPeakD : Outport  Port=13
  MotCtrlMotCurrAdcPeakE : Outport  Port=14
  MotCtrlMotCurrAdcPeakF : Outport  Port=15
  MotCtrlMotCurrSnsrOffs1 : Outport  Port=16
  MotCtrlMotCurrSnsrOffs2 : Outport  Port=17
  MotCtrlAdc0ScanGroup2Ref1 : Outport  Port=18
  MotCtrlAdc0SelfDiag0 : Outport  Port=19
  MotCtrlAdc0SelfDiag2 : Outport  Port=20
  MotCtrlAdc0SelfDiag4 : Outport  Port=21
  wires:
  Unity Scaling Factor/1 -> Convert Adc Results/2
  Unity Scaling Factor1/1 -> Convert Adc Results1/2
  Unity Scaling Factor2/1 -> Convert Adc Results2/2
  Unity Scaling Factor3/1 -> Convert Adc Results3/2
  Unity Scaling Factor4/1 -> Convert Adc Results4/2
  Unity Scaling Factor5/1 -> Convert Adc Results5/2
  Unity Scaling Factor6/1 -> Convert Adc Results6/2
  Unity Scaling Factor7/1 -> Convert Adc Results7/2
  Unity Scaling Factor8/1 -> Convert Adc Results8/2
  Unity Scaling Factor9/1 -> Convert Adc Results9/2
  Unity Scaling Factor10/1 -> Convert Adc Results10/2
  Unity Scaling Factor11/1 -> Convert Adc Results11/2
  Unity Scaling Factor13/1 -> Convert Adc Results13/2
  Unity Scaling Factor14/1 -> Convert Adc Results14/2
  Unity Scaling Factor19/1 -> Convert Adc Results19/2
  Unity Scaling Factor20/1 -> Convert Adc Results20/2
  Unity Scaling Factor21/1 -> Convert Adc Results21/2
  Convert Adc Results/1 -> MotCtrlMotCurrAdcVlyA/1
  Convert Adc Results1/1 -> MotCtrlMotCurrAdcVlyB/1
  Convert Adc Results2/1 -> MotCtrlMotCurrAdcVlyC/1
  Convert Adc Results3/1 -> MotCtrlMotCurrAdcVlyD/1
  Convert Adc Results4/1 -> MotCtrlMotCurrAdcVlyE/1
  Convert Adc Results5/1 -> MotCtrlMotCurrAdcVlyF/1
  Convert Adc Results6/1 -> MotCtrlMotCurrAdcPeakA/1
  Convert Adc Results7/1 -> MotCtrlMotCurrAdcPeakB/1
  Convert Adc Results8/1 -> MotCtrlMotCurrAdcPeakC/1
  Convert Adc Results9/1 -> MotCtrlMotCurrAdcPeakD/1
  Convert Adc Results10/1 -> MotCtrlMotCurrAdcPeakE/1
  Convert Adc Results11/1 -> MotCtrlMotCurrAdcPeakF/1
  Convert Adc Results13/1 -> MotCtrlMotCurrSnsrOffs1/1
  Convert Adc Results14/1 -> MotCtrlMotCurrSnsrOffs2/1
  Convert Adc Results19/1 -> MotCtrlAdc0SelfDiag0/1
  Convert Adc Results20/1 -> MotCtrlAdc0SelfDiag2/1
  Convert Adc Results21/1 -> MotCtrlAdc0SelfDiag4/1
  RegInpADCD0DR00/1 -> Bitwise Operator/1, Shift Arithmetic/1
  RegInpADCD0DR02/1 -> Shift Arithmetic1/1, Bitwise Operator1/1
  RegInpADCD0DR04/1 -> Bitwise Operator2/1, Shift Arithmetic2/1
  RegInpADCD0DR06/1 -> Shift Arithmetic3/1, Bitwise Operator3/1
  RegInpADCD0DR08/1 -> Bitwise Operator4/1, Shift Arithmetic4/1
  RegInpADCD0DR10/1 -> Bitwise Operator5/1, Shift Arithmetic5/1
  RegInpADCD0DR12/1 -> Bitwise Operator6/1, Shift Arithmetic6/1
  RegInpADCD0DR14/1 -> Bitwise Operator7/1, Shift Arithmetic7/1
  RegInpADCD0DR16/1 -> Bitwise Operator8/1, Shift Arithmetic8/1
  RegInpADCD0DR18/1 -> Bitwise Operator9/1, Shift Arithmetic9/1
  RegInpADCD0DR20/1 -> Bitwise Operator10/1, Shift Arithmetic10/1
  RegInpADCD0DR22/1 -> Bitwise Operator11/1, Shift Arithmetic11/1
  Shift Arithmetic11/1 -> Convert Adc Results21/1
  Bitwise Operator11/1 -> Convert Adc Results20/1
  Shift Arithmetic10/1 -> Convert Adc Results19/1
  Bitwise Operator10/1 -> Terminator5/1
  Shift Arithmetic9/1 -> Terminator4/1
  Unity Scaling Factor15/1 -> Convert Adc Results15/2
  Convert Adc Results15/1 -> MotCtrlAdc0ScanGroup3Ref0/1
  Bitwise Operator/1 -> Convert Adc Results15/1
  Bitwise Operator7/1 -> Convert Adc Results11/1
  Shift Arithmetic6/1 -> Convert Adc Results10/1
  Bitwise Operator6/1 -> Convert Adc Results9/1
  Shift Arithmetic5/1 -> Convert Adc Results8/1
  Bitwise Operator5/1 -> Convert Adc Results7/1
  Shift Arithmetic4/1 -> Convert Adc Results6/1
  Shift Arithmetic/1 -> Convert Adc Results/1
  Bitwise Operator1/1 -> Convert Adc Results1/1
  Shift Arithmetic1/1 -> Convert Adc Results2/1
  Bitwise Operator2/1 -> Convert Adc Results3/1
  Shift Arithmetic2/1 -> Convert Adc Results4/1
  Bitwise Operator3/1 -> Convert Adc Results5/1
  Unity Scaling Factor16/1 -> Convert Adc Results16/2
  Convert Adc Results16/1 -> MotCtrlAdc0ScanGroup3Ref1/1
  Shift Arithmetic3/1 -> Convert Adc Results16/1
  Unity Scaling Factor17/1 -> Convert Adc Results17/2
  Convert Adc Results17/1 -> MotCtrlAdc0ScanGroup2Ref0/1
  Bitwise Operator4/1 -> Convert Adc Results17/1
  Unity Scaling Factor18/1 -> Convert Adc Results18/2
  Convert Adc Results18/1 -> MotCtrlAdc0ScanGroup2Ref1/1
  Shift Arithmetic7/1 -> Convert Adc Results13/1
  Bitwise Operator8/1 -> Convert Adc Results14/1
  Shift Arithmetic8/1 -> Convert Adc Results18/1
  Bitwise Operator9/1 -> Terminator1/1

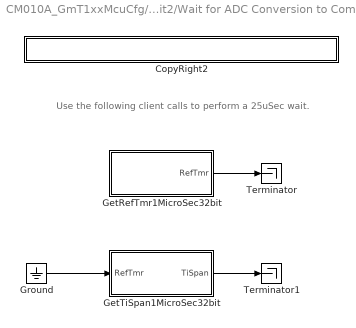
== system CM010A_GmT1xxMcuCfg/GmT1xxMcuCfg/GmT1xxMcuCfgInit2/Wait for ADC Conversion to Complete ==
  note: Use the following client calls to perform a 25uSec wait.
  CopyRight2 : Subsystem  Description=|  mask(Copyright Information){none=on}
      | Copyright info block.                                               
      |                                                                     
      | Place copyright information at the top of every subsystem in design.
      mask prompts: none "No parameters"
      mask help: Place copyright information at the top of every subsystem in design.
      mask Display:
      | NxtrConf = 'Nexteer Confidential';
      | 
      | sys = bdroot; %handle for the current model ("system")
      | first = get_param(sys,'Created');
      | first = first(end-3:end);  %year is last four digits
      | 
      | last = get_param(sys,'LastModifiedDate');
      | if isempty(last)
      |     last = datestr(now,'yyyy');
      | else
      |     last = last(end-3:end);
      | end
      | 
      | if strcmp(first,last)
      |     fprintf('%s -- Copyright %s Nexteer',NxtrConf,first)
      | else
      |     fprintf('%s -- %s%s- %s Nexteer',NxtrConf,char(169),first,last)
      | end
  GetRefTmr1MicroSec32bit : Subsystem  TreatAsAtomicUnit=on
  GetTiSpan1MicroSec32bit : Subsystem  TreatAsAtomicUnit=on
  Ground : Ground
  Terminator : Terminator
  Terminator1 : Terminator
  wires:
  GetRefTmr1MicroSec32bit/1(RefTmr) -> Terminator/1
  GetTiSpan1MicroSec32bit/1(TiSpan) -> Terminator1/1
  Ground/1 -> GetTiSpan1MicroSec32bit/1(RefTmr)

== system CM010A_GmT1xxMcuCfg/GmT1xxMcuCfg/GmT1xxMcuCfgInit3/CopyRight2 ==

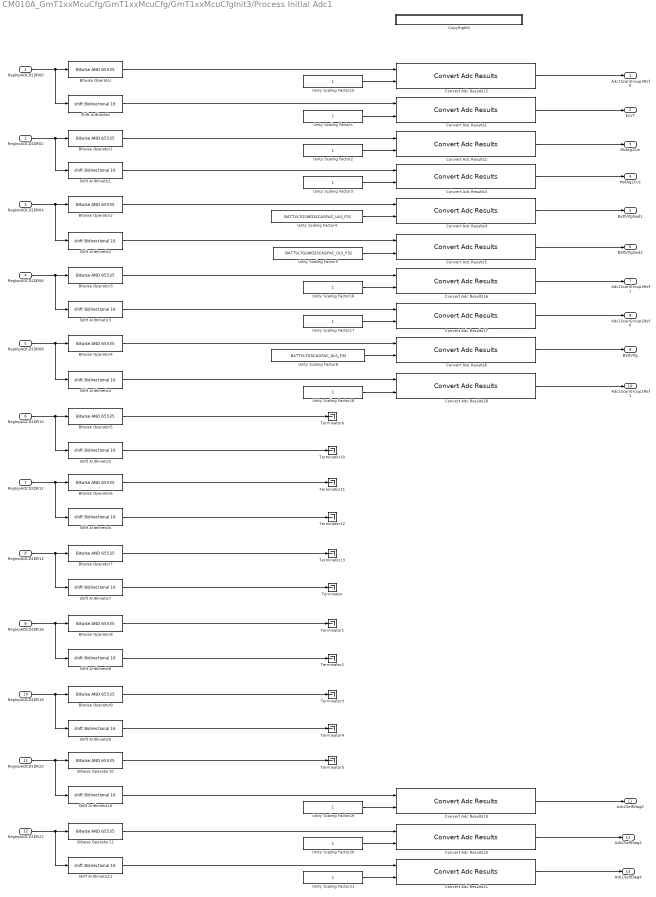
== system CM010A_GmT1xxMcuCfg/GmT1xxMcuCfg/GmT1xxMcuCfgInit3/Process Initial Adc1 ==
  RegInpADCD1DR00 : Inport  OutDataTypeStr=uint32
  RegInpADCD1DR02 : Inport  Port=2  OutDataTypeStr=uint32
  RegInpADCD1DR04 : Inport  Port=3  OutDataTypeStr=uint32
  RegInpADCD1DR06 : Inport  Port=4  OutDataTypeStr=uint32
  RegInpADCD1DR08 : Inport  Port=5  OutDataTypeStr=uint32
  RegInpADCD1DR10 : Inport  Port=6  OutDataTypeStr=uint32
  RegInpADCD1DR12 : Inport  Port=7  OutDataTypeStr=uint32
  RegInpADCD1DR14 : Inport  Port=8  OutDataTypeStr=uint32
  RegInpADCD1DR16 : Inport  Port=9  OutDataTypeStr=uint32
  RegInpADCD1DR18 : Inport  Port=10  OutDataTypeStr=uint32
  RegInpADCD1DR20 : Inport  Port=11  OutDataTypeStr=uint32
  RegInpADCD1DR22 : Inport  Port=12  OutDataTypeStr=uint32
  Bitwise Operator{,1..11} (12 alike) : simulink/Logic and Bit Operations/Bitwise Operator  logicop=AND  UseBitMask=on  BitMask=65535  BitMaskRealWorld=Stored Integer
  Convert Adc Results{1..6,15..21} (13 alike) : CM010A_GmT1xxMcuCfg_ModelLibrary/Convert Adc Results
  CopyRight2 : Subsystem  Description=|  mask(Copyright Information){none=on}
      | Copyright info block.                                               
      |                                                                     
      | Place copyright information at the top of every subsystem in design.
      mask prompts: none "No parameters"
      mask help: Place copyright information at the top of every subsystem in design.
      mask Display:
      | NxtrConf = 'Nexteer Confidential';
      | 
      | sys = bdroot; %handle for the current model ("system")
      | first = get_param(sys,'Created');
      | first = first(end-3:end);  %year is last four digits
      | 
      | last = get_param(sys,'LastModifiedDate');
      | if isempty(last)
      |     last = datestr(now,'yyyy');
      | else
      |     last = last(end-3:end);
      | end
      | 
      | if strcmp(first,last)
      |     fprintf('%s -- Copyright %s Nexteer',NxtrConf,first)
      | else
      |     fprintf('%s -- %s%s- %s Nexteer',NxtrConf,char(169),first,last)
      | end
  Shift Arithmetic{,1..11} (12 alike) : ArithShift  BitShiftNumber=16
  Terminator{,1..6,10..13} (11 alike) : Terminator
  Unity Scaling Factor{1..3,15..21} (10 alike) : Constant  OutDataTypeStr=single
  Unity Scaling Factor4 : Constant  Value=BATTVLTGSWD1SCAGFAC_ULS_F32  OutDataTypeStr=single
  Unity Scaling Factor5 : Constant  Value=BATTVLTGSWD2SCAGFAC_ULS_F32  OutDataTypeStr=single
  Unity Scaling Factor6 : Constant  Value=BATTVLTGSCAGFAC_ULS_F32  OutDataTypeStr=single
  Adc1ScanGroup3Ref0 : Outport
  EcuT : Outport  Port=2
  MotAg2Sin : Outport  Port=3
  MotAg2Cos : Outport  Port=4
  BattVltgSwd1 : Outport  Port=5
  BattVltgSwd2 : Outport  Port=6
  Adc1ScanGroup3Ref1 : Outport  Port=7
  Adc1ScanGroup2Ref0 : Outport  Port=8
  BattVltg : Outport  Port=9
  Adc1ScanGroup2Ref1 : Outport  Port=10
  Adc1SelfDiag0 : Outport  Port=11
  Adc1SelfDiag2 : Outport  Port=12
  Adc1SelfDiag4 : Outport  Port=13
  wires:
  Convert Adc Results21/1 -> Adc1SelfDiag4/1
  Convert Adc Results20/1 -> Adc1SelfDiag2/1
  Convert Adc Results19/1 -> Adc1SelfDiag0/1
  Convert Adc Results6/1 -> BattVltg/1
  Convert Adc Results5/1 -> BattVltgSwd2/1
  Convert Adc Results4/1 -> BattVltgSwd1/1
  Convert Adc Results3/1 -> MotAg2Cos/1
  Convert Adc Results2/1 -> MotAg2Sin/1
  Convert Adc Results1/1 -> EcuT/1
  Unity Scaling Factor21/1 -> Convert Adc Results21/2
  Unity Scaling Factor20/1 -> Convert Adc Results20/2
  Unity Scaling Factor19/1 -> Convert Adc Results19/2
  Unity Scaling Factor6/1 -> Convert Adc Results6/2
  Unity Scaling Factor5/1 -> Convert Adc Results5/2
  Unity Scaling Factor4/1 -> Convert Adc Results4/2
  Unity Scaling Factor3/1 -> Convert Adc Results3/2
  Unity Scaling Factor2/1 -> Convert Adc Results2/2
  Unity Scaling Factor1/1 -> Convert Adc Results1/2
  RegInpADCD1DR00/1 -> Bitwise Operator/1, Shift Arithmetic/1
  RegInpADCD1DR02/1 -> Bitwise Operator1/1, Shift Arithmetic1/1
  RegInpADCD1DR04/1 -> Bitwise Operator2/1, Shift Arithmetic2/1
  RegInpADCD1DR06/1 -> Bitwise Operator3/1, Shift Arithmetic3/1
  RegInpADCD1DR08/1 -> Bitwise Operator4/1, Shift Arithmetic4/1
  RegInpADCD1DR10/1 -> Bitwise Operator5/1, Shift Arithmetic5/1
  RegInpADCD1DR12/1 -> Bitwise Operator6/1, Shift Arithmetic6/1
  RegInpADCD1DR14/1 -> Bitwise Operator7/1, Shift Arithmetic7/1
  RegInpADCD1DR16/1 -> Bitwise Operator8/1, Shift Arithmetic8/1
  RegInpADCD1DR18/1 -> Bitwise Operator9/1, Shift Arithmetic9/1
  RegInpADCD1DR20/1 -> Bitwise Operator10/1, Shift Arithmetic10/1
  RegInpADCD1DR22/1 -> Bitwise Operator11/1, Shift Arithmetic11/1
  Shift Arithmetic11/1 -> Convert Adc Results21/1
  Bitwise Operator11/1 -> Convert Adc Results20/1
  Shift Arithmetic10/1 -> Convert Adc Results19/1
  Bitwise Operator10/1 -> Terminator5/1
  Bitwise Operator9/1 -> Terminator3/1
  Shift Arithmetic9/1 -> Terminator4/1
  Bitwise Operator8/1 -> Terminator1/1
  Shift Arithmetic8/1 -> Terminator2/1
  Shift Arithmetic7/1 -> Terminator/1
  Shift Arithmetic5/1 -> Terminator10/1
  Bitwise Operator6/1 -> Terminator11/1
  Shift Arithmetic6/1 -> Terminator12/1
  Bitwise Operator7/1 -> Terminator13/1
  Unity Scaling Factor15/1 -> Convert Adc Results15/2
  Convert Adc Results15/1 -> Adc1ScanGroup3Ref0/1
  Unity Scaling Factor16/1 -> Convert Adc Results16/2
  Convert Adc Results16/1 -> Adc1ScanGroup3Ref1/1
  Unity Scaling Factor17/1 -> Convert Adc Results17/2
  Convert Adc Results17/1 -> Adc1ScanGroup2Ref0/1
  Unity Scaling Factor18/1 -> Convert Adc Results18/2
  Convert Adc Results18/1 -> Adc1ScanGroup2Ref1/1
  Bitwise Operator/1 -> Convert Adc Results15/1
  Shift Arithmetic/1 -> Convert Adc Results1/1
  Bitwise Operator1/1 -> Convert Adc Results2/1
  Shift Arithmetic1/1 -> Convert Adc Results3/1
  Bitwise Operator2/1 -> Convert Adc Results4/1
  Shift Arithmetic2/1 -> Convert Adc Results5/1
  Bitwise Operator3/1 -> Convert Adc Results16/1
  Shift Arithmetic3/1 -> Convert Adc Results17/1
  Bitwise Operator4/1 -> Convert Adc Results6/1
  Shift Arithmetic4/1 -> Convert Adc Results18/1
  Bitwise Operator5/1 -> Terminator6/1
